simulink model "STM32MPU9250"  (R2018b)
settings: Solver=FixedStepAuto  StartTime=0.0  StopTime=10.0  FixedStep=0.01  RelTol=1e-3  EnableMultiTasking=on
values from neighbouring files (symbols this model uses):
  Data = uint8(Data)    [MPU9250.m]
  Read = uint8(59:59+19)    [MPU9250.m]
libraries: simulink x5, mbedblockslib x2
settings Model: ExtModeTrigDuration=10  Creator=Syed Imtiaz Ali Shah  LastModifiedBy=Syed Imtiaz Ali Shah
settings OptimizationCC: EnhancedBackFolding=on  PassReuseOutputArgsAs=Individual arguments  MaxStackSize=64  OptimizeBlockOrder=speed  DifferentSizesBufferReuse=on  OptimizationCustomize=off
settings DebuggingCC: ParameterTunabilityLossMsg=error
settings HardwareCC: ProdBitPerPointer=32  ProdBitPerSizeT=32  ProdBitPerPtrDiffT=32  ProdLargestAtomicInteger=Long  ProdLargestAtomicFloat=Double  ProdWordSize=32  ProdHWDeviceType=ARM Compatible->ARM Cortex
settings SFSimCC: SimCustomHeaderCode="#include \"store.h\""  SimUserSources=store.c  MATLABDynamicMemAlloc=off
settings RTWCC: SystemTargetFile=ert.tlc  HardwareBoard=STM32 Nucleo F103RB  TemplateMakefile=ert_default_tmf  GenerateReport=on  RTWUseSimCustomCode=on  CustomHeaderCode="#include \"store.h\""  CustomSource=store.c  Toolchain=GNU Tools for ARM Embedded Processors  IncludeHyperlinkInReport=on  LaunchReport=on  GenerateTraceInfo=on  GenerateTraceReport=on  GenerateTraceReportSl=on  GenerateTraceReportSf=on  GenerateTraceReportEml=on
settings CodeAppCC: ForceParamTrailComments=on  IgnoreCustomStorageClasses=off  OperatorAnnotations=on  SimulinkDataObjDesc=on  SFDataObjDesc=on  InsertBlockDesc=on

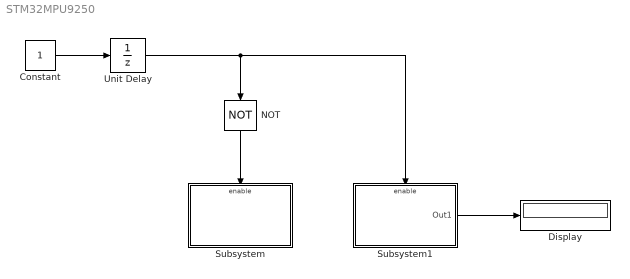
== system STM32MPU9250 ==
  Constant : Constant  SampleTime=-1
  Display : Display
  NOT : Logic  Operator=NOT  AllPortsSameDT=off  OutDataTypeStr=boolean
  Subsystem : Subsystem
  Subsystem1 : Subsystem
  Unit Delay : UnitDelay  SampleTime=-1
  wires:
  Constant/1 -> Unit Delay/1
  Unit Delay/1 -> Subsystem1/Enable, NOT/1
  NOT/1 -> Subsystem/Enable
  Subsystem1/1(Out1) -> Display/1

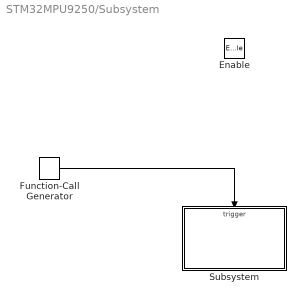
== system STM32MPU9250/Subsystem ==
  Enable : EnablePort
  Function-Call Generator : simulink/Ports & Subsystems/Function-Call Generator  sample_time=1  numberOfIterations=1
  Subsystem : Subsystem
  wires:
  Function-Call Generator/1 -> Subsystem/Trigger

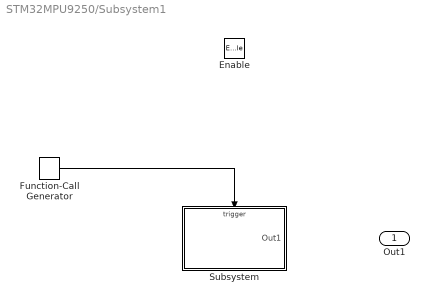
== system STM32MPU9250/Subsystem1 ==
  Enable : EnablePort
  Function-Call Generator : simulink/Ports & Subsystems/Function-Call Generator  sample_time=1  numberOfIterations=1
  Subsystem : Subsystem
  Out1 : Outport
  wires:
  ? -> Out1/1
  Function-Call Generator/1 -> Subsystem/Trigger

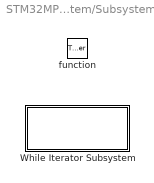
== system STM32MPU9250/Subsystem/Subsystem ==
  function : TriggerPort  TriggerType=function-call  VariantControl=Variant
  While Iterator Subsystem : Subsystem  TreatAsAtomicUnit=on

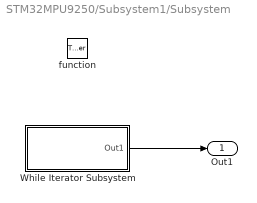
== system STM32MPU9250/Subsystem1/Subsystem ==
  function : TriggerPort  TriggerType=function-call  VariantControl=Variant
  While Iterator Subsystem : Subsystem  TreatAsAtomicUnit=on
  Out1 : Outport
  wires:
  While Iterator Subsystem/1(Out1) -> Out1/1

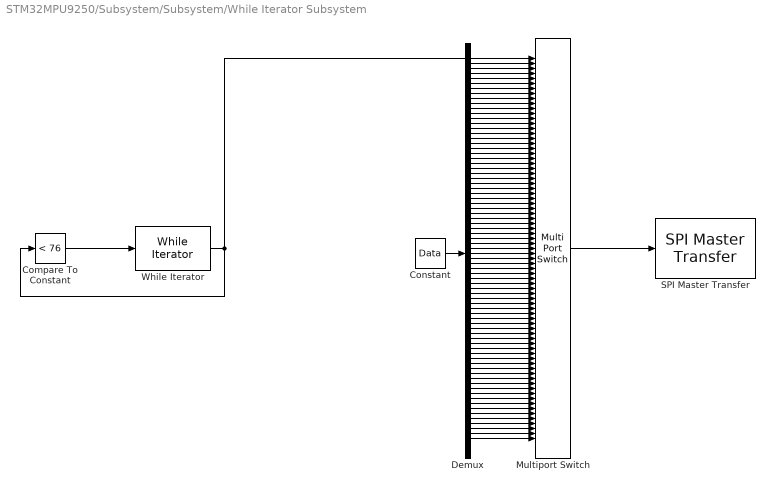
== system STM32MPU9250/Subsystem/Subsystem/While Iterator Subsystem ==
  Compare To Constant : simulink/Logic and Bit Operations/Compare To Constant  relop=<  const=76  OutDataTypeStr=boolean
  Constant : Constant  Value=Data
  Demux : Demux  Outputs=76
  Multiport Switch : MultiPortSwitch  Inputs=76
  SPI Master Transfer : mbedblockslib/SPI Master Transfer  SPIModule=0  Mode=Master  BusSpeed=uint32( 1000000 )  Pin=D4  FirstBitToTransfer=Most significant bit (MSB)  ClockMode=3  BlockFunction=Transfer  RegisterAddress=0  OutputDataType=int8  OutputDataLength=1  UseCustomSSPin=Explicit GPIO calls  ActiveLowSSPin=Active low
      settings: SourceProductName=Simulink Coder Support Package for BBC microbit Board  SourceProductBaseCode=MICROBIT
  While Iterator : WhileIterator  MaxIters=84  WhileBlockType=do-while  ShowIterationPort=on
  wires:
  Compare To Constant/1 -> While Iterator/1
  While Iterator/1 -> Multiport Switch/1, Compare To Constant/1
  Demux/1 -> Multiport Switch/2
  Demux/2 -> Multiport Switch/3
  Demux/3 -> Multiport Switch/4
  Demux/4 -> Multiport Switch/5
  Demux/5 -> Multiport Switch/6
  Demux/6 -> Multiport Switch/7
  Demux/7 -> Multiport Switch/8
  Demux/8 -> Multiport Switch/9
  Demux/9 -> Multiport Switch/10
  Demux/10 -> Multiport Switch/11
  Demux/11 -> Multiport Switch/12
  Demux/12 -> Multiport Switch/13
  Demux/13 -> Multiport Switch/14
  Demux/14 -> Multiport Switch/15
  Demux/15 -> Multiport Switch/16
  Demux/16 -> Multiport Switch/17
  Demux/17 -> Multiport Switch/18
  Demux/18 -> Multiport Switch/19
  Demux/19 -> Multiport Switch/20
  Demux/20 -> Multiport Switch/21
  Demux/21 -> Multiport Switch/22
  Demux/22 -> Multiport Switch/23
  Demux/23 -> Multiport Switch/24
  Demux/24 -> Multiport Switch/25
  Demux/25 -> Multiport Switch/26
  Demux/26 -> Multiport Switch/27
  Demux/27 -> Multiport Switch/28
  Demux/28 -> Multiport Switch/29
  Demux/29 -> Multiport Switch/30
  Demux/30 -> Multiport Switch/31
  Demux/31 -> Multiport Switch/32
  Demux/32 -> Multiport Switch/33
  Demux/33 -> Multiport Switch/34
  Demux/34 -> Multiport Switch/35
  Demux/35 -> Multiport Switch/36
  Demux/36 -> Multiport Switch/37
  Demux/37 -> Multiport Switch/38
  Demux/38 -> Multiport Switch/39
  Demux/39 -> Multiport Switch/40
  Demux/40 -> Multiport Switch/41
  Demux/41 -> Multiport Switch/42
  Demux/42 -> Multiport Switch/43
  Demux/43 -> Multiport Switch/44
  Demux/44 -> Multiport Switch/45
  Demux/45 -> Multiport Switch/46
  Demux/46 -> Multiport Switch/47
  Demux/47 -> Multiport Switch/48
  Demux/48 -> Multiport Switch/49
  Demux/49 -> Multiport Switch/50
  Demux/50 -> Multiport Switch/51
  Demux/51 -> Multiport Switch/52
  Demux/52 -> Multiport Switch/53
  Demux/53 -> Multiport Switch/54
  Demux/54 -> Multiport Switch/55
  Demux/55 -> Multiport Switch/56
  Demux/56 -> Multiport Switch/57
  Demux/57 -> Multiport Switch/58
  Demux/58 -> Multiport Switch/59
  Demux/59 -> Multiport Switch/60
  Demux/60 -> Multiport Switch/61
  Demux/61 -> Multiport Switch/62
  Demux/62 -> Multiport Switch/63
  Demux/63 -> Multiport Switch/64
  Demux/64 -> Multiport Switch/65
  Demux/65 -> Multiport Switch/66
  Demux/66 -> Multiport Switch/67
  Demux/67 -> Multiport Switch/68
  Demux/68 -> Multiport Switch/69
  Demux/69 -> Multiport Switch/70
  Demux/70 -> Multiport Switch/71
  Demux/71 -> Multiport Switch/72
  Demux/72 -> Multiport Switch/73
  Constant/1 -> Demux/1
  Multiport Switch/1 -> SPI Master Transfer/1
  Demux/73 -> Multiport Switch/74
  Demux/74 -> Multiport Switch/75
  Demux/75 -> Multiport Switch/76
  Demux/76 -> Multiport Switch/77

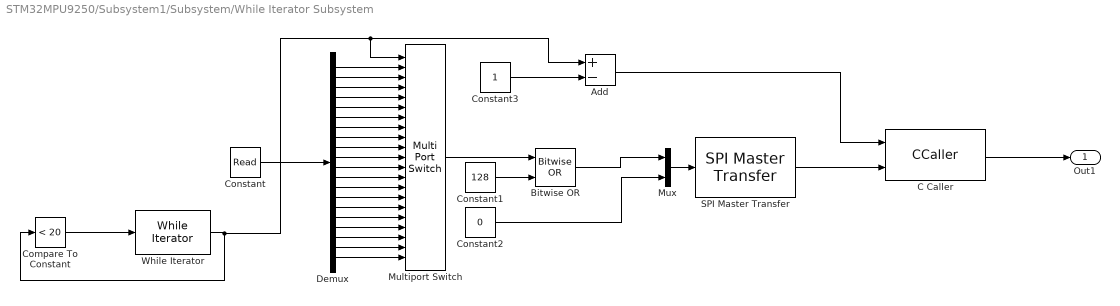
== system STM32MPU9250/Subsystem1/Subsystem/While Iterator Subsystem ==
  Add : Sum  Inputs=+-
  Bitwise OR : simulink/Logic and Bit Operations/Bitwise Operator  logicop=OR  UseBitMask=off  NumInputPorts=2  BitMask=bin2dec('11011001')  BitMaskRealWorld=Stored Integer
  C Caller : CCaller  FunctionName=storeIt  PortSpecificationStruct="%)30     .    R 0   8    (     @         %    \"     ,    !     0         %  0 \"0    $    V    07)G3F%M90  4&]R=$YA;64 4V-O<&4     26YD97@     5'EP90      4VEZ90         .    ,     8    (    !          %    \"     $    #     0         0  , ;W5T  X    P    !@    @    $          4    (     0    ,    !         !   P!O=70 #@   #@    &    \"     0         !0    @    !    !@    $         $     8   !/=71P=70   X    X    !@    @    &          4    (     0    $    !          D    (               .    .     8    (    !          %    \"     $    %     0         0    !0   '5I;G0X    #@   #     &    \"     0         !0    @    !     0    $         $  ! #$    .    .     8    (    !          %    \"     $    %     0         0    !0   &EN9&5X    #@   #@    &    \"     0         !0    @    !    !0    $         $     4   !I;F1E>     X    X    !@    @    $          4    (     0    4    !         !     %    26YP=70    .    .     8    (    !@         %    \"     $    !     0         )    \"               #@   #@    &    \"     0         !0    @    !    !0    $         $     4   !I;G0S,@    X    P    !@    @    $          4    (     0    $    !         !   0 Q    #@   #@    &    \"     0         !0    @    !    !0    $         $     4   !I;G!U=     X    X    !@    @    $          4    (     0    4    !         !     %    :6YP=70    .    .     8    (    !          %    \"     $    %     0         0    !0   $EN<'5T    #@   #@    &    \"     8         !0    @    !     0    $         \"0    @           #P/PX    X    !@    @    $          4    (     0    4    !         !     %    =6EN=#@    .    ,     8    (    !          %    \"     $    !     0         0  $ ,0"
  Compare To Constant : simulink/Logic and Bit Operations/Compare To Constant  relop=<  const=20  OutDataTypeStr=boolean
  Constant : Constant  Value=Read
  Constant1 : Constant  Value=128  OutDataTypeStr=uint8
  Constant2 : Constant  Value=0  OutDataTypeStr=uint8
  Constant3 : Constant  OutDataTypeStr=uint8
  Demux : Demux  Outputs=20
  Multiport Switch : MultiPortSwitch  Inputs=20
  Mux : Mux  Inputs=2
  SPI Master Transfer : mbedblockslib/SPI Master Transfer  SPIModule=0  Mode=Master  BusSpeed=uint32( 1000000 )  Pin=D4  FirstBitToTransfer=Most significant bit (MSB)  ClockMode=3  BlockFunction=Transfer  RegisterAddress=0  OutputDataType=int8  OutputDataLength=1  UseCustomSSPin=Explicit GPIO calls  ActiveLowSSPin=Active low
      settings: SourceProductName=Simulink Coder Support Package for BBC microbit Board  SourceProductBaseCode=MICROBIT
  While Iterator : WhileIterator  MaxIters=84  WhileBlockType=do-while  ShowIterationPort=on
  Out1 : Outport
  wires:
  While Iterator/1 -> Add/1, Multiport Switch/1, Compare To Constant/1
  Compare To Constant/1 -> While Iterator/1
  Demux/1 -> Multiport Switch/2
  Demux/2 -> Multiport Switch/3
  Demux/3 -> Multiport Switch/4
  Demux/4 -> Multiport Switch/5
  Demux/5 -> Multiport Switch/6
  Demux/6 -> Multiport Switch/7
  Demux/7 -> Multiport Switch/8
  Demux/8 -> Multiport Switch/9
  Demux/9 -> Multiport Switch/10
  Demux/10 -> Multiport Switch/11
  Demux/11 -> Multiport Switch/12
  Demux/12 -> Multiport Switch/13
  Demux/13 -> Multiport Switch/14
  Demux/14 -> Multiport Switch/15
  Demux/15 -> Multiport Switch/16
  Demux/16 -> Multiport Switch/17
  Demux/17 -> Multiport Switch/18
  Demux/18 -> Multiport Switch/19
  Demux/19 -> Multiport Switch/20
  Demux/20 -> Multiport Switch/21
  Constant/1 -> Demux/1
  Multiport Switch/1 -> Bitwise OR/1
  Constant1/1 -> Bitwise OR/2
  Mux/1 -> SPI Master Transfer/1
  Bitwise OR/1 -> Mux/1
  Constant2/1 -> Mux/2
  Constant3/1 -> Add/2
  Add/1 -> C Caller/1
  SPI Master Transfer/1 -> C Caller/2
  C Caller/1 -> Out1/1
